simulink model "qp_Sim"  (R2020a)
settings: Solver=VariableStepAuto  StartTime=0.0  StopTime=10.0  RelTol=1e-3
settings Model: Creator=niran  LastModifiedBy=niranjan.bhujel

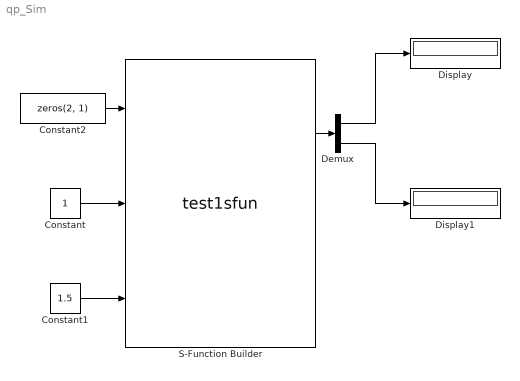
== system qp_Sim ==
  Constant : Constant
  Constant1 : Constant  Value=1.5
  Constant2 : Constant  Value=zeros(2, 1)
  Demux : Demux  Outputs=2
  Display : Display
  Display1 : Display
  S-Function Builder : S-Function  InitFcn=try, set_param(gcb,'FunctionName','test1sfun'), end  FunctionName=test1sfun  SFunctionModules=test1sfun_wrapper test1 test1_EVAL_CODE test1_EVAL_CODE_Call BLASReplacement Bounds Constraints Flipper Indexlist LAPACKReplacement Matrices MessageHandling Options OQPinterface QProblem QProblemB SolutionAnalysis SparseSolver SQProblem SQProblemSchur SubjectTo Utils  SFunctionDeploymentMode=off  EnableBusSupport=off  mask(S-Function Builder){}
      mask help: Simulink:masks:SFunctionBuilder_MD
      mask init:
      | val = [[.9  0.75 0.75 1 1 .9 .9 1]',[1 1 0.75 0.75 .9 .9 1 .9]'];try , sys = get_param(gcb,'SfunBuilderFcnName');if isempty(sys), sys = get_param(gcb,'FunctionName'); end,catch, sys = get_param(gcb,'FunctionName'); end
      settings: CopyFcn=set_param(gcbh,'LinkStatus','none')  PreSaveFcn=try, set_param(gcb,'FunctionName','test1sfun'), end  OpenFcn=sfunctionwizard(gcbh)
      mask Display: plot(val(:,1),val(:,2)),disp(sys), port_label('input',1,'xGuess'), port_label('input',2,'a'), port_label('input',3,'b'), port_label('output',1,'xOpt_VAL'), port_label('output',2,'Obj_VAL')
  wires:
  Constant/1 -> S-Function Builder/2
  Constant1/1 -> S-Function Builder/3
  Constant2/1 -> S-Function Builder/1
  S-Function Builder/1 -> Demux/1
  Demux/1 -> Display/1
  Demux/2 -> Display1/1
